simulink model "lqr_controller"  (R2023a)
settings: Solver=VariableStepAuto  StartTime=0.0  StopTime=10.0  RelTol=1e-3
values from neighbouring files (symbols this model uses):
  A_m = [0 1 0; M_alpha 0 M_alpha/V; -(F-Drag+N_alpha)/m 0 -N_alpha/(m*V)]    [AutopilotDesign.m]
  B_m = [0; M_delta; Tc/m]    [AutopilotDesign.m]
  C_m = diag([1 1 1])    [AutopilotDesign.m]
  D_m = [0;0;0]    [AutopilotDesign.m]
  K_1 = K(1)    [cost_function.m]
  K_2 = K(2)    [cost_function.m]
  K_3 = K(3)    [cost_function.m]
undefined symbols (not defined in the file or in its folder): Earth, WGS84
libraries: aerolibfltsims x2, aerolibtransform2 x1
settings Model: Creator=ramonadevi  LastModifiedBy=ramonadevi

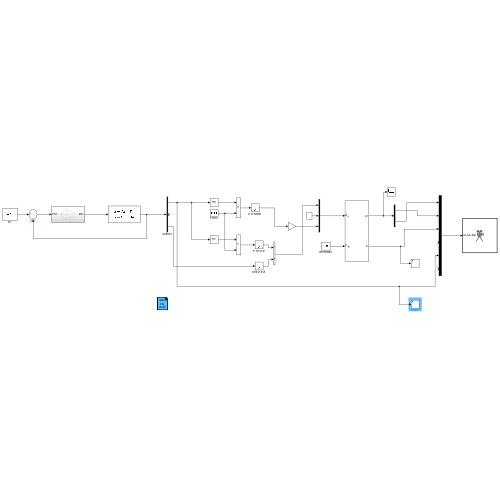
[thumbnail: Simulink's stored preview of the top-level diagram]
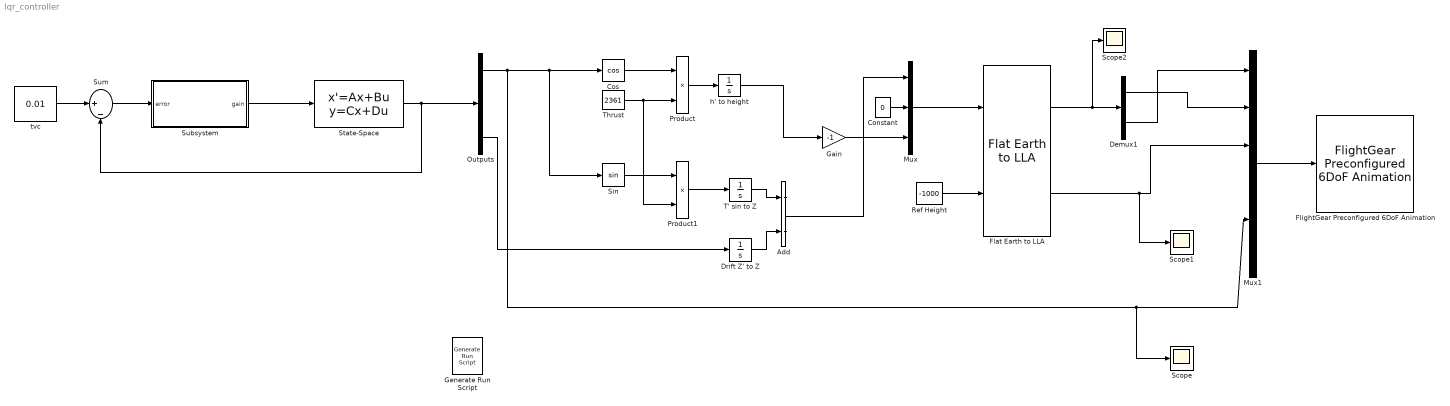
== system lqr_controller ==
  Add : Sum
  Constant : Constant  Value=0
  Cos : Trigonometry  Operator=cos
  Demux1 : Demux  Outputs=2
  Drift Z' to Z : Integrator
  Flat Earth to LLA : aerolibtransform2/Flat Earth to LLA  units=Metric (MKS)  ptype=Earth (WGS84)  F=1/298.257223563  R=6378137  refPosPort=off  LL0=[0 10]  psi=0
  FlightGear Preconfigured 6DoF Animation : aerolibfltsims/FlightGear Preconfigured 6DoF Animation  xFlightGearVersion=v2019.1  DestinationIpAddress=127.0.0.1  DestinationPort=5502  SampleTime=1/30  packetVersion=24
  Gain : Gain  Gain=-1
  Generate Run Script : aerolibfltsims/Generate Run Script  Architecture=Mac  dataFlow=Send  GeometryModelName=c172p  AirportId=KSFO  RunwayId=10L  InitialAltitude=7224  InitialHeading=113  OffsetDistance=4.72  OffsetAzimuth=0  InstallScenery=off  DisableShaders=off  OriginAddress=127.0.0.1  DestinationPort=5502  OriginPort=5505  LocalAddress=127.0.0.1  OutputFileName=runfg.bat  FlightGearBaseDirectory=/Applications/FlightGear.app
  Mux : Mux  Inputs=3
  Mux1 : Mux  Inputs=6
  Outputs : Demux  Outputs=3
  Product : Product
  Product1 : Product
  Ref Height : Constant  Value=-1000
  Scope : Scope
  Scope1 : Scope
  Scope2 : Scope
  Sin : Trigonometry
  State-Space : StateSpace  A=A_m  B=B_m  C=C_m  D=D_m  InitialCondition=[0.2;0;0]
  Subsystem : Subsystem
  Sum : Sum  Inputs=|+-
  T' sin to Z : Integrator
  Thrust : Constant  Value=2361
  h' to height : Integrator
  tvc : Constant  Value=0.01
  wires:
  tvc/1 -> Sum/1
  State-Space/1 -> Outputs/1, Sum/2
  Sum/1 -> Subsystem/1(error)
  Subsystem/1(gain) -> State-Space/1
  Outputs/1 -> Scope/1, Mux1/5, Sin/1, Cos/1
  Cos/1 -> Product/1
  Thrust/1 -> Product1/2, Product/2
  Sin/1 -> Product1/1
  Outputs/3 -> Drift Z' to Z/1
  Product/1 -> h' to height/1
  Product1/1 -> T' sin to Z/1
  Drift Z' to Z/1 -> Add/2
  T' sin to Z/1 -> Add/1
  Gain/1 -> Mux/3
  h' to height/1 -> Gain/1
  Add/1 -> Mux/1
  Constant/1 -> Mux/2
  Mux/1 -> Flat Earth to LLA/1
  Ref Height/1 -> Flat Earth to LLA/2
  Flat Earth to LLA/1 -> Scope2/1, Demux1/1
  Demux1/1 -> Mux1/2
  Demux1/2 -> Mux1/1
  Flat Earth to LLA/2 -> Scope1/1, Mux1/3
  Mux1/1 -> FlightGear Preconfigured 6DoF Animation/1

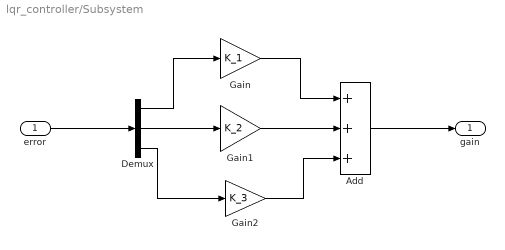
== system lqr_controller/Subsystem ==
  error : Inport
  Add : Sum  Inputs=+++
  Demux : Demux  Outputs=3
  Gain : Gain  Gain=K_1
  Gain1 : Gain  Gain=K_2
  Gain2 : Gain  Gain=K_3
  gain : Outport
  wires:
  Add/1 -> gain/1
  error/1 -> Demux/1
  Gain/1 -> Add/1
  Gain2/1 -> Add/3
  Demux/2 -> Gain1/1
  Demux/3 -> Gain2/1
  Gain1/1 -> Add/2
  Demux/1 -> Gain/1
